simulink model "vm_verification"  (Simulink 6.6)
settings: Solver=VariableStepDiscrete  StartTime=0.0  StopTime=10000  RelTol=1e-3
libraries: xbsIndex_r4 x6, simulink x4
settings Model: Creator=lcrockett  LastModifiedBy=lcrockett
settings OptimizationCC: InlineParams=on

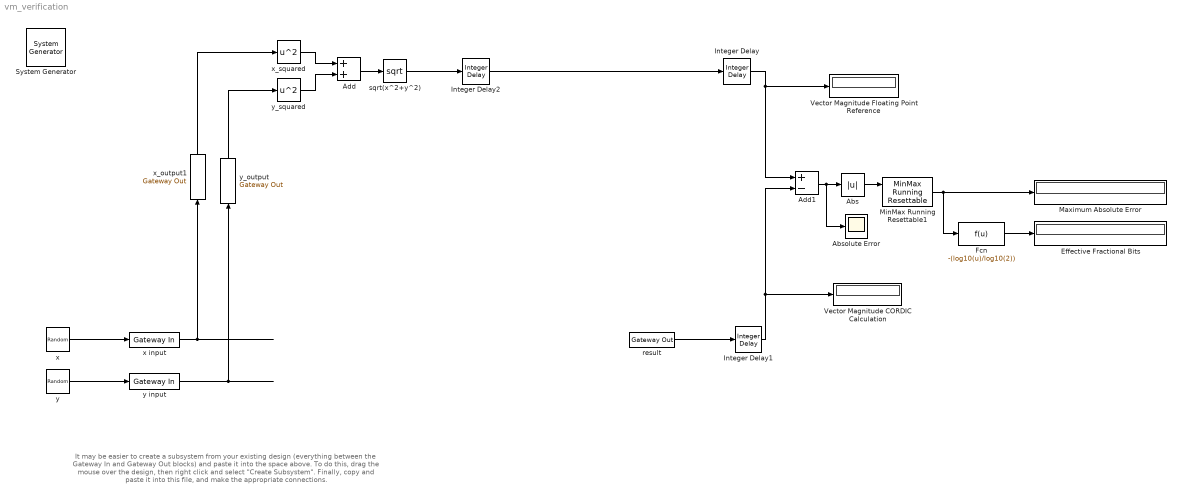
== system vm_verification ==
  note: It may be easier to create a subsystem from your existing design (everything between the Gateway In and Gateway Out blocks)
      | and paste it into the space above. To do this, drag the mouse over the design, then right click and select "Create Subsystem".
      | Finally, copy and paste it into this file, and make the appropriate connections.
  " System Generator" : xbsIndex_r4/ System Generator  Tag=genX  SystemSampleTime=-1  xilinxfamily=virtex2p  part=xc2vp30  speed=-7  package=ff896  synthesis_tool=XST  clock_wrapper=Clock Enables  directory=./netlist  testbench=off  simulink_period=1  sysclk_period=25  dcm_input_clock_period=100  incr_netlist=off  trim_vbits=Everywhere in SubSystem  dbl_ovrd=According to Block Masks  core_generation=According to Block Masks  run_coregen=off  deprecated_control=off  eval_field=0  block_type=sysgen
      settings: block_version=10.1.2
  Abs : Abs
  Absolute Error : Scope
  Add : Sum  OutScaling=2^-10
  Add1 : Sum  Inputs=+-  OutScaling=2^-10
  Effective Fractional Bits : Display
      settings: Format=decimal (Stored Integer)
  Fcn : Fcn  Expr=-(log10(u)/log10(2))
  Integer Delay : simulink/Discrete/Integer Delay  vinit=0.0  samptime=-1  NumDelays=1
  Integer Delay1 : simulink/Discrete/Integer Delay  vinit=0.0  samptime=-1  NumDelays=1
  Integer Delay2 : simulink/Discrete/Integer Delay  vinit=0.0  samptime=-1  NumDelays=2
  Maximum Absolute Error : Display
      settings: Format=long_e
  MinMax Running Resettable1 : simulink/Math Operations/MinMax Running Resettable  SystemSampleTime=-1  Function=max  vinit=0.0
  Vector Magnitude CORDIC Calculation : Display
  Vector Magnitude Floating Point Reference : Display
  result : xbsIndex_r4/Gateway Out  hdl_port=on  timing_constraint=None  locs_specified=off  LOCs={}  block_type=gatewayout
      settings: infoedit="Gateway out block.  Converts Xilinx fixed point inputs into ouputs of type Simulink integer, double, or fixed point.<P><P>Hardware notes:  In hardware these blocks become top level output ports or are discarded, depending on how they are configured."  block_version=10.1.2
  sqrt(x^2+y^2) : Math  Operator=sqrt  SaturateOnIntegerOverflow=on
  x : UniformRandomNumber  Minimum=-0.5  Maximum=0.5  Seed=1324  SampleTime=1
  x input : xbsIndex_r4/Gateway In  arith_type="Signed  (2's comp)"  n_bits=16  bin_pt=13  quantization="Round  (unbiased: +/- Inf)"  overflow=Saturate  period=1  dbl_ovrd=off  timing_constraint=None  locs_specified=off  LOCs={}  block_type=gatewayin
      settings: infoedit="Gateway in block.  Converts inputs of type Simulink integer, double and fixed point to  Xilinx fixed point type.<P><P>Hardware notes:  In hardware these blocks become top level input ports."  block_version=10.1.2
  x_output1 : xbsIndex_r4/Gateway Out  Orientation=up  hdl_port=on  timing_constraint=None  locs_specified=off  LOCs={}  block_type=gatewayout
      settings: infoedit="Gateway out block.  Converts Xilinx fixed point inputs into ouputs of type Simulink integer, double, or fixed point.<P><P>Hardware notes:  In hardware these blocks become top level output ports or are discarded, depending on how they are configured."  block_version=10.1.2
  x_squared : Math  Operator=square  SaturateOnIntegerOverflow=on
  y : UniformRandomNumber  Minimum=-0.5  Maximum=0.5  Seed=4679  SampleTime=1
  y input : xbsIndex_r4/Gateway In  arith_type="Signed  (2's comp)"  n_bits=16  bin_pt=13  quantization="Round  (unbiased: +/- Inf)"  overflow=Saturate  period=1  dbl_ovrd=off  timing_constraint=None  locs_specified=off  LOCs={}  block_type=gatewayin
      settings: infoedit="Gateway in block.  Converts inputs of type Simulink integer, double and fixed point to  Xilinx fixed point type.<P><P>Hardware notes:  In hardware these blocks become top level input ports."  block_version=10.1.2
  y_output : xbsIndex_r4/Gateway Out  Orientation=up  hdl_port=on  timing_constraint=None  locs_specified=off  LOCs={}  block_type=gatewayout
      settings: infoedit="Gateway out block.  Converts Xilinx fixed point inputs into ouputs of type Simulink integer, double, or fixed point.<P><P>Hardware notes:  In hardware these blocks become top level output ports or are discarded, depending on how they are configured."  block_version=10.1.2
  y_squared : Math  Operator=square  SaturateOnIntegerOverflow=on
  wires:
  x/1 -> x input/1
  y/1 -> y input/1
  x_squared/1 -> Add/1
  y_squared/1 -> Add/2
  Add/1 -> sqrt(x^2+y^2)/1
  sqrt(x^2+y^2)/1 -> Integer Delay2/1
  Add1/1 -> Abs/1, Absolute Error/1
  Abs/1 -> MinMax Running Resettable1/1
  MinMax Running Resettable1/1 -> Maximum Absolute Error/1, Fcn/1
  result/1 -> Integer Delay1/1
  Integer Delay2/1 -> Integer Delay/1
  ? -> result/1
  x input/1 -> x_output1/1
  y input/1 -> y_output/1
  Fcn/1 -> Effective Fractional Bits/1
  x_output1/1 -> x_squared/1
  y_output/1 -> y_squared/1
  Integer Delay/1 -> Add1/1, Vector Magnitude Floating Point Reference/1
  Integer Delay1/1 -> Add1/2, Vector Magnitude CORDIC Calculation/1
